simulink model "SubsistemaConRetardo"  (R2024b)
settings: Solver=VariableStepAuto  StartTime=0.0  StopTime=40000  RelTol=1e-3
undefined symbols (not defined in the file): n, p1, p2, p3, Vi
libraries: slpidlib x2, eeAlternativeControllers x1
settings Model: Creator=HP  LastModifiedBy=HP

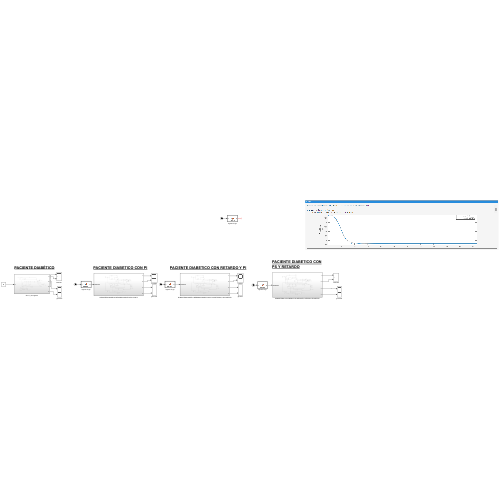
[thumbnail: Simulink's stored preview of the top-level diagram]
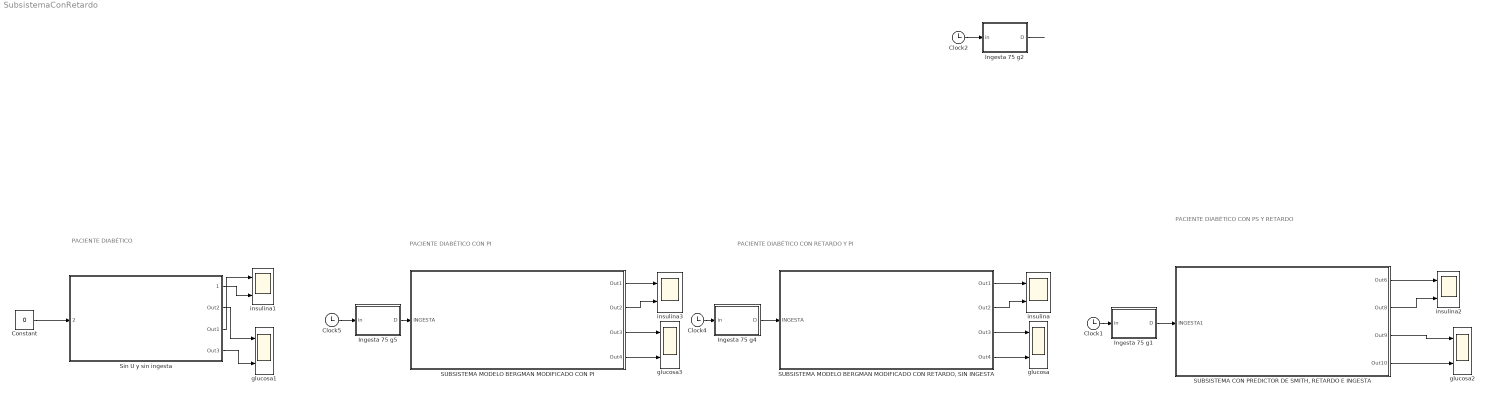
== system SubsistemaConRetardo ==
  note: PACIENTE DIABÉTICO
  note: PACIENTE DIABÉTICO CON RETARDO Y PI
  note: PACIENTE DIABÉTICO CON PI
  note: PACIENTE DIABÉTICO CON PS Y RETARDO
  Clock{1..2,4..5} (4 alike) : Clock
  Constant : Constant  Value=0
  Ingesta 75 g1 : MATLAB Function  TreatAsAtomicUnit=on
  Ingesta 75 g2 : MATLAB Function  TreatAsAtomicUnit=on
  Ingesta 75 g4 : MATLAB Function  TreatAsAtomicUnit=on
  Ingesta 75 g5 : MATLAB Function  TreatAsAtomicUnit=on
  "SUBSISTEMA CON PREDICTOR DE SMITH, RETARDO E INGESTA" : Subsystem
  SUBSISTEMA MODELO BERGMAN MODIFICADO CON PI : Subsystem
  "SUBSISTEMA MODELO BERGMAN MODIFICADO CON RETARDO, SIN INGESTA" : Subsystem
  Sin U y sin ingesta : Subsystem
  glucosa{,1..3} (4 alike) : Scope  NumInputPorts=2
  insulina{,1..3} (4 alike) : Scope  NumInputPorts=2
  wires:
  "SUBSISTEMA MODELO BERGMAN MODIFICADO CON RETARDO, SIN INGESTA"/1(Out1) -> insulina/1
  "SUBSISTEMA MODELO BERGMAN MODIFICADO CON RETARDO, SIN INGESTA"/2(Out2) -> insulina/2
  "SUBSISTEMA MODELO BERGMAN MODIFICADO CON RETARDO, SIN INGESTA"/3(Out3) -> glucosa/1
  "SUBSISTEMA MODELO BERGMAN MODIFICADO CON RETARDO, SIN INGESTA"/4(Out4) -> glucosa/2
  "SUBSISTEMA CON PREDICTOR DE SMITH, RETARDO E INGESTA"/4(Out10) -> glucosa2/2
  "SUBSISTEMA CON PREDICTOR DE SMITH, RETARDO E INGESTA"/2(Out8) -> insulina2/2
  "SUBSISTEMA CON PREDICTOR DE SMITH, RETARDO E INGESTA"/1(Out6) -> insulina2/1
  "SUBSISTEMA CON PREDICTOR DE SMITH, RETARDO E INGESTA"/3(Out9) -> glucosa2/1
  SUBSISTEMA MODELO BERGMAN MODIFICADO CON PI/3(Out3) -> glucosa3/1
  SUBSISTEMA MODELO BERGMAN MODIFICADO CON PI/1(Out1) -> insulina3/1
  SUBSISTEMA MODELO BERGMAN MODIFICADO CON PI/2(Out2) -> insulina3/2
  SUBSISTEMA MODELO BERGMAN MODIFICADO CON PI/4(Out4) -> glucosa3/2
  Sin U y sin ingesta/1(1) -> insulina1/2
  Sin U y sin ingesta/2(Out2) -> glucosa1/1
  Sin U y sin ingesta/3(Out1) -> insulina1/1
  Sin U y sin ingesta/4(Out3) -> glucosa1/2
  Constant/1 -> Sin U y sin ingesta/1(2)
  Ingesta 75 g2/1(D) -> ?
  Clock2/1 -> Ingesta 75 g2/1(in)
  Clock4/1 -> Ingesta 75 g4/1(in)
  Ingesta 75 g4/1(D) -> "SUBSISTEMA MODELO BERGMAN MODIFICADO CON RETARDO, SIN INGESTA"/1(INGESTA)
  Clock5/1 -> Ingesta 75 g5/1(in)
  Ingesta 75 g5/1(D) -> SUBSISTEMA MODELO BERGMAN MODIFICADO CON PI/1(INGESTA)
  Ingesta 75 g1/1(D) -> "SUBSISTEMA CON PREDICTOR DE SMITH, RETARDO E INGESTA"/1(INGESTA1)
  Clock1/1 -> Ingesta 75 g1/1(in)

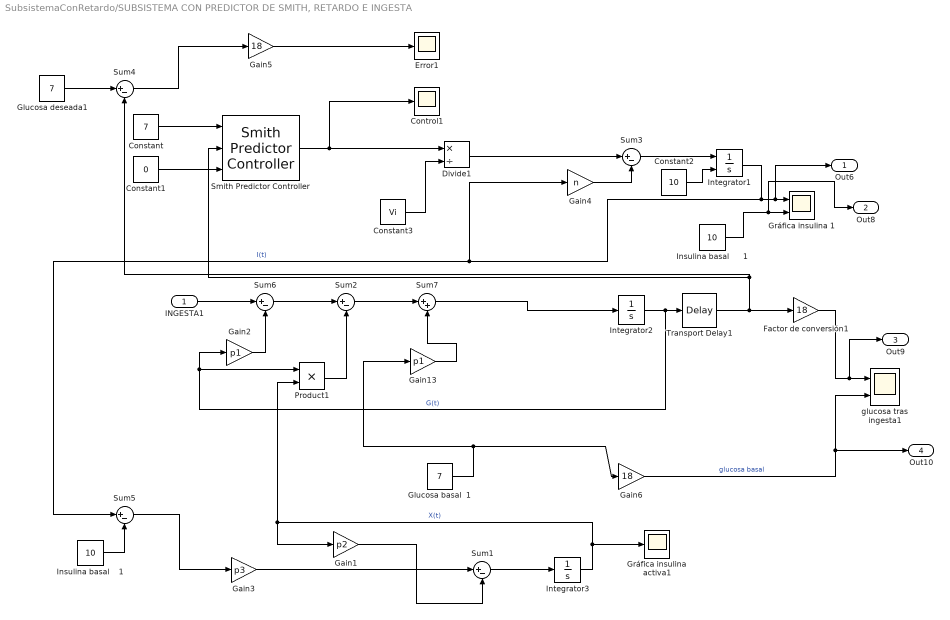
== system SubsistemaConRetardo/SUBSISTEMA CON PREDICTOR DE SMITH, RETARDO E INGESTA ==
  INGESTA1 : Inport
  Constant : Constant  Value=7
  Constant1 : Constant  Value=0
  Constant2 : Constant  Value=10
  Constant3 : Constant  Value=Vi
  Control1 : Scope
  Divide1 : Product  Inputs=*/
  Error1 : Scope
  Factor de conversión1 : Gain  Gain=18
  Gain1 : Gain  Gain=p2
  Gain13 : Gain  Gain=p1
  Gain2 : Gain  Gain=p1
  Gain3 : Gain  Gain=p3
  Gain4 : Gain  Gain=n
  Gain5 : Gain  Gain=18
  Gain6 : Gain  Gain=18
  Glucosa basal  1 : Constant  Value=7
  Glucosa deseada1 : Constant  Value=7
  Gráfica insulina 1 : Scope  NumInputPorts=2
  Gráfica insulina activa1 : Scope
  Insulina basal      1 : Constant  Value=10
  Insulina basal    1 : Constant  Value=10
  Integrator1 : Integrator  InitialConditionSource=external
  Integrator2 : Integrator  InitialCondition=7
  Integrator3 : Integrator
  Product1 : Product
  Smith Predictor Controller : eeAlternativeControllers/Smith Predictor Controller  Kp=-0.3195  Ki=-0.3195/2998.95  x0=0  B=5  A=0  numd=[8.979]  dend=[1, 0.6205, 0.1686]  d=900  Ts=1
  Sum{1..6} (6 alike) : Sum  Inputs=|+-
  Sum7 : Sum  Inputs=|++
  Transport Delay1 : TransportDelay  DelayTime=900  InitialOutput=7
  glucosa tras ingesta1 : Scope  NumInputPorts=2
  Out6 : Outport
  Out8 : Outport  Port=2
  Out9 : Outport  Port=3
  Out10 : Outport  Port=4
  wires:
  Gain13/1 -> Sum7/2
  INGESTA1/1 -> Sum6/1
  Gain2/1 -> Sum6/2
  Sum6/1 -> Sum2/1
  Insulina basal      1/1 -> Out8/1, Gráfica insulina 1/2
  Gain4/1 -> Sum3/2
  Integrator1/1 -> Out6/1, Gráfica insulina 1/1, Sum5/1, Gain4/1  "I(t)"
  Gain5/1 -> Error1/1
  Factor de conversión1/1 -> Out9/1, glucosa tras ingesta1/1
  Sum7/1 -> Integrator2/1
  Sum5/1 -> Gain3/1
  Sum3/1 -> Integrator1/1
  Sum4/1 -> Gain5/1
  Product1/1 -> Sum2/2
  Constant3/1 -> Divide1/2
  Integrator3/1 -> Product1/2, Gain1/1, Gráfica insulina activa1/1  "X(t)"
  Gain6/1 -> Out10/1, glucosa tras ingesta1/2  "glucosa basal"
  Glucosa deseada1/1 -> Sum4/1
  Integrator2/1 -> Gain2/1, Product1/1, Transport Delay1/1  "G(t)"
  Glucosa basal  1/1 -> Gain13/1, Gain6/1
  Divide1/1 -> Sum3/1
  Constant2/1 -> Integrator1/2
  Sum2/1 -> Sum7/1
  Smith Predictor Controller/1 -> Control1/1, Divide1/1
  Gain1/1 -> Sum1/2
  Constant1/1 -> Smith Predictor Controller/3
  Insulina basal    1/1 -> Sum5/2
  Gain3/1 -> Sum1/1
  Constant/1 -> Smith Predictor Controller/1
  Sum1/1 -> Integrator3/1
  Transport Delay1/1 -> Smith Predictor Controller/2, Sum4/2, Factor de conversión1/1

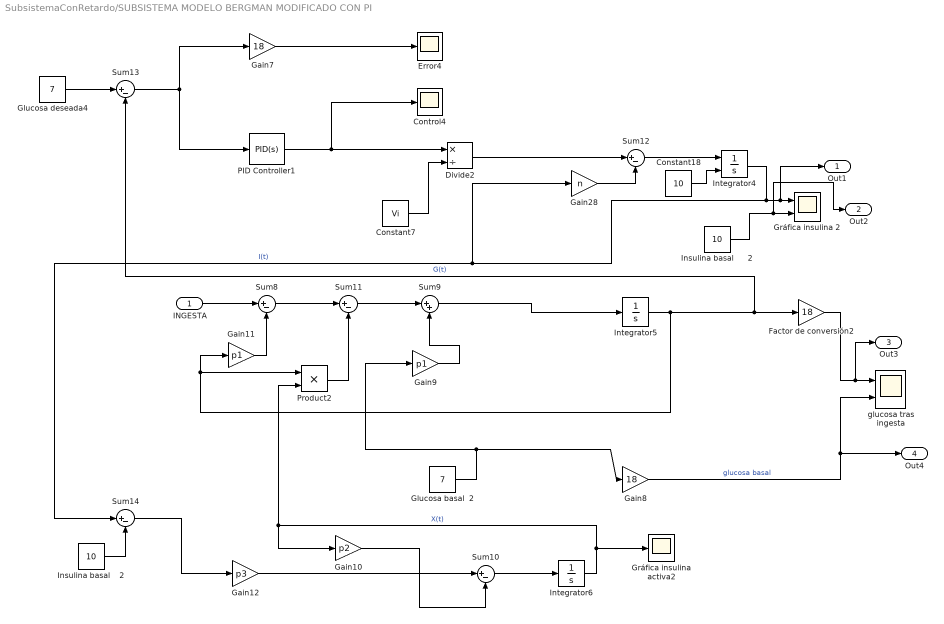
== system SubsistemaConRetardo/SUBSISTEMA MODELO BERGMAN MODIFICADO CON PI ==
  INGESTA : Inport
  Constant18 : Constant  Value=10
  Constant7 : Constant  Value=Vi
  Control4 : Scope
  Divide2 : Product  Inputs=*/
  Error4 : Scope
  Factor de conversión2 : Gain  Gain=18
  Gain10 : Gain  Gain=p2
  Gain11 : Gain  Gain=p1
  Gain12 : Gain  Gain=p3
  Gain28 : Gain  Gain=n
  Gain7 : Gain  Gain=18
  Gain8 : Gain  Gain=18
  Gain9 : Gain  Gain=p1
  Glucosa basal  2 : Constant  Value=7
  Glucosa deseada4 : Constant  Value=7
  Gráfica insulina 2 : Scope  NumInputPorts=2
  Gráfica insulina activa2 : Scope
  Insulina basal      2 : Constant  Value=10
  Insulina basal    2 : Constant  Value=10
  Integrator4 : Integrator  InitialConditionSource=external
  Integrator5 : Integrator  InitialCondition=7
  Integrator6 : Integrator
  PID Controller1 : slpidlib/PID Controller  Controller=PID  Form=Parallel  TimeDomain=Continuous-time  UseExternalTs=off  SampleTime=-1  IntegratorMethod=Forward Euler  FilterMethod=Forward Euler  ControllerParametersSource=internal  P=-0.3195  I=-0.3195/2998.95  UseKiTs=off  D=0  UseExternalDerivativeSource=off  N=10  UseFilter=on  TunerSelectOption=Transfer Function Based (PID Tuner App)  InitialConditionSource=internal  InitialConditionForIntegrator=0  InitialConditionForFilter=0  DifferentiatorICPrevScaledInput=0  ExternalReset=none  TrackingMode=off  Kt=1  LimitOutput=off  SatLimitsSource=internal  UpperSaturationLimit=inf  LowerSaturationLimit=-inf  LinearizeAsGain=on  AntiWindupMode=none  Kb=1  LimitIntegrator=off  UpperIntegratorSaturationLimit=inf  LowerIntegratorSaturationLimit=-inf  POutMin=[]  POutMax=[]  IOutMin=[]  IOutMax=[]  DOutMin=[]  DOutMax=[]  NOutMin=[]  NOutMax=[]  SumOutMin=[]  SumOutMax=[]  SaturationOutMin=[]  SaturationOutMax=[]  PParamMin=[]  PParamMax=[]  IParamMin=[]  IParamMax=[]  DParamMin=[]  DParamMax=[]  NParamMin=[]  NParamMax=[]  KbParamMin=[]  KbParamMax=[]  KtParamMin=[]  KtParamMax=[]  KbOutMin=[]  KbOutMax=[]  KtOutMin=[]  KtOutMax=[]  IntegratorOutMin=[]  IntegratorOutMax=[]  FilterOutMin=[]  FilterOutMax=[]  SumI1OutMin=[]  SumI1OutMax=[]  SumI2OutMin=[]  SumI2OutMax=[]  SumI3OutMin=[]  SumI3OutMax=[]  SumI4OutMin=[]  SumI4OutMax=[]  SumDOutMin=[]  SumDOutMax=[]  DifferentiatorOutMin=[]  DifferentiatorOutMax=[]  FilterDiffOutCoefMin=[]  FilterDiffOutCoefMax=[]  ReciprocalOutMin=[]  ReciprocalOutMax=[]  SumDenOutMin=[]  SumDenOutMax=[]  SumNumOutMin=[]  SumNumOutMax=[]  DivideOutMin=[]  DivideOutMax=[]  UdiffTsProdOutMin=[]  UdiffTsProdOutMax=[]  NTsProdOutMin=[]  NTsProdOutMax=[]  UintegralTsProdOutMin=[]  UintegralTsProdOutMax=[]  UngainTsProdOutMin=[]  UngainTsProdOutMax=[]  ClampingZeroOutDataTypeStr=Inherit: Inherit via back propagation  ClampingZeroOutMin=[]  ClampingZeroOutMax=[]  FilterDenConstantOutDataTypeStr=Inherit: Inherit via back propagation  FilterDenConstantOutMin=[]  FilterDenConstantOutMax=[]  PCopyOutDataTypeStr=Inherit: Inherit via back propagation  PCopyOutMin=[]  PCopyOutMax=[]  NCopyOutDataTypeStr=Inherit: Inherit via back propagation  NCopyOutMin=[]  NCopyOutMax=[]  IntegratorContinuousStateAttributes=''  IntegratorStateMustResolveToSignalObject=off  IntegratorRTWStateStorageClass=Auto  FilterContinuousStateAttributes=''  FilterStateMustResolveToSignalObject=off  FilterRTWStateStorageClass=Auto  ParallelPVariant=InternalParameters  IdealPVariant=Disabled  IVariant=InternalParameters  DVariant=InternalParameters  IntegratorVariant=Continuous  SatVariant=Disabled  AWVariant=Passthrough  PCopyVariant=Disabled  TRVariant=Disabled  FdbkBlocksVariant=Forward  IdealPFdbkVariant=Disabled  SatFdbkVariant=Disabled  DerivativeFilterVariant=ContFilter  NVariant=InternalParameters  NCopyVariant=Disabled  FilterICVariant=InternalICsFilter  IntegratorICVariant=InternalICs  ExternalResetVariant=Disabled  TRSumVariant=Passthrough  SumFdbkVariant=Disabled  SumVariant=Sum_PID  TsampFilterVariant=InternalTs  TsampNgainVariant=Passthrough  TsampIntegralVariant=Disabled_SignalSpec  ExternalSaturationOutDataTypeStr=Inherit: Same as second input  DerivativeSourceVariant=ErrorSignal  PreIntVariant=InternalPreInt
  Product2 : Product
  Sum{8,10..14} (6 alike) : Sum  Inputs=|+-
  Sum9 : Sum  Inputs=|++
  glucosa tras ingesta : Scope  NumInputPorts=2
  Out1 : Outport
  Out2 : Outport  Port=2
  Out3 : Outport  Port=3
  Out4 : Outport  Port=4
  wires:
  Integrator6/1 -> Product2/2, Gain10/1, Gráfica insulina activa2/1  "X(t)"
  Factor de conversión2/1 -> Out3/1, glucosa tras ingesta/1
  Sum11/1 -> Sum9/1
  Sum12/1 -> Integrator4/1
  Integrator5/1 -> Sum13/2, Factor de conversión2/1, Gain11/1, Product2/1  "G(t)"
  Gain8/1 -> glucosa tras ingesta/2, Out4/1  "glucosa basal"
  Sum14/1 -> Gain12/1
  Insulina basal      2/1 -> Out2/1, Gráfica insulina 2/2
  Integrator4/1 -> Out1/1, Gráfica insulina 2/1, Sum14/1, Gain28/1  "I(t)"
  Gain9/1 -> Sum9/2
  Glucosa basal  2/1 -> Gain9/1, Gain8/1
  Gain12/1 -> Sum10/1
  Glucosa deseada4/1 -> Sum13/1
  Constant7/1 -> Divide2/2
  Sum9/1 -> Integrator5/1
  Gain10/1 -> Sum10/2
  Product2/1 -> Sum11/2
  Gain28/1 -> Sum12/2
  Sum10/1 -> Integrator6/1
  Sum8/1 -> Sum11/1
  Sum13/1 -> PID Controller1/1, Gain7/1
  Insulina basal    2/1 -> Sum14/2
  Gain11/1 -> Sum8/2
  Gain7/1 -> Error4/1
  Divide2/1 -> Sum12/1
  PID Controller1/1 -> Control4/1, Divide2/1
  Constant18/1 -> Integrator4/2
  INGESTA/1 -> Sum8/1

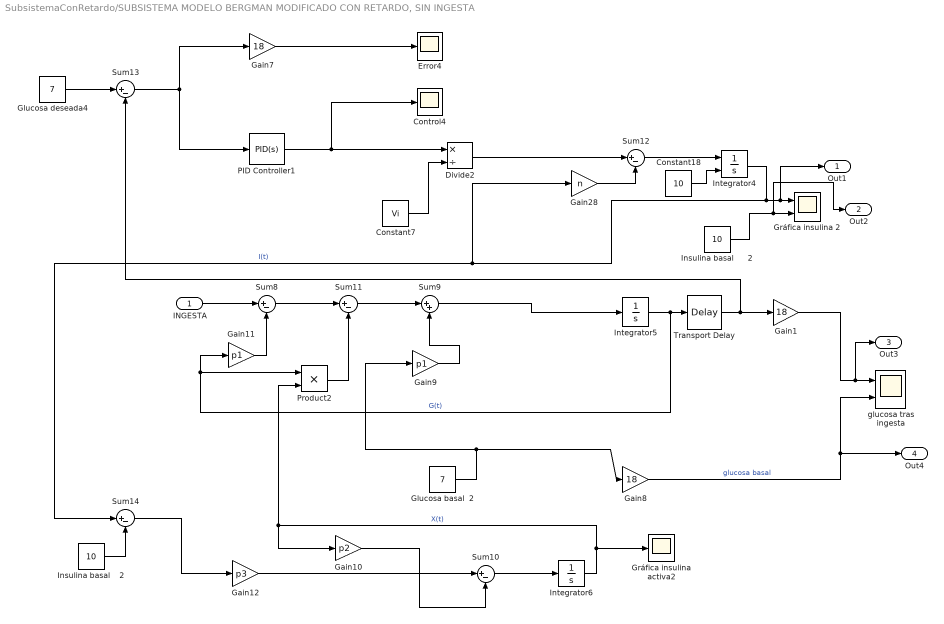
== system SubsistemaConRetardo/SUBSISTEMA MODELO BERGMAN MODIFICADO CON RETARDO, SIN INGESTA ==
  INGESTA : Inport
  Constant18 : Constant  Value=10
  Constant7 : Constant  Value=Vi
  Control4 : Scope
  Divide2 : Product  Inputs=*/
  Error4 : Scope
  Gain1 : Gain  Gain=18
  Gain10 : Gain  Gain=p2
  Gain11 : Gain  Gain=p1
  Gain12 : Gain  Gain=p3
  Gain28 : Gain  Gain=n
  Gain7 : Gain  Gain=18
  Gain8 : Gain  Gain=18
  Gain9 : Gain  Gain=p1
  Glucosa basal  2 : Constant  Value=7
  Glucosa deseada4 : Constant  Value=7
  Gráfica insulina 2 : Scope  NumInputPorts=2
  Gráfica insulina activa2 : Scope
  Insulina basal      2 : Constant  Value=10
  Insulina basal    2 : Constant  Value=10
  Integrator4 : Integrator  InitialConditionSource=external
  Integrator5 : Integrator  InitialCondition=7
  Integrator6 : Integrator
  PID Controller1 : slpidlib/PID Controller  Controller=PID  Form=Parallel  TimeDomain=Continuous-time  UseExternalTs=off  SampleTime=-1  IntegratorMethod=Forward Euler  FilterMethod=Forward Euler  ControllerParametersSource=internal  P=-0.3195  I=-0.3195/2998.95  UseKiTs=off  D=0  UseExternalDerivativeSource=off  N=10  UseFilter=on  TunerSelectOption=Transfer Function Based (PID Tuner App)  InitialConditionSource=internal  InitialConditionForIntegrator=0  InitialConditionForFilter=0  DifferentiatorICPrevScaledInput=0  ExternalReset=none  TrackingMode=off  Kt=1  LimitOutput=off  SatLimitsSource=internal  UpperSaturationLimit=inf  LowerSaturationLimit=-inf  LinearizeAsGain=on  AntiWindupMode=none  Kb=1  LimitIntegrator=off  UpperIntegratorSaturationLimit=inf  LowerIntegratorSaturationLimit=-inf  POutMin=[]  POutMax=[]  IOutMin=[]  IOutMax=[]  DOutMin=[]  DOutMax=[]  NOutMin=[]  NOutMax=[]  SumOutMin=[]  SumOutMax=[]  SaturationOutMin=[]  SaturationOutMax=[]  PParamMin=[]  PParamMax=[]  IParamMin=[]  IParamMax=[]  DParamMin=[]  DParamMax=[]  NParamMin=[]  NParamMax=[]  KbParamMin=[]  KbParamMax=[]  KtParamMin=[]  KtParamMax=[]  KbOutMin=[]  KbOutMax=[]  KtOutMin=[]  KtOutMax=[]  IntegratorOutMin=[]  IntegratorOutMax=[]  FilterOutMin=[]  FilterOutMax=[]  SumI1OutMin=[]  SumI1OutMax=[]  SumI2OutMin=[]  SumI2OutMax=[]  SumI3OutMin=[]  SumI3OutMax=[]  SumI4OutMin=[]  SumI4OutMax=[]  SumDOutMin=[]  SumDOutMax=[]  DifferentiatorOutMin=[]  DifferentiatorOutMax=[]  FilterDiffOutCoefMin=[]  FilterDiffOutCoefMax=[]  ReciprocalOutMin=[]  ReciprocalOutMax=[]  SumDenOutMin=[]  SumDenOutMax=[]  SumNumOutMin=[]  SumNumOutMax=[]  DivideOutMin=[]  DivideOutMax=[]  UdiffTsProdOutMin=[]  UdiffTsProdOutMax=[]  NTsProdOutMin=[]  NTsProdOutMax=[]  UintegralTsProdOutMin=[]  UintegralTsProdOutMax=[]  UngainTsProdOutMin=[]  UngainTsProdOutMax=[]  ClampingZeroOutDataTypeStr=Inherit: Inherit via back propagation  ClampingZeroOutMin=[]  ClampingZeroOutMax=[]  FilterDenConstantOutDataTypeStr=Inherit: Inherit via back propagation  FilterDenConstantOutMin=[]  FilterDenConstantOutMax=[]  PCopyOutDataTypeStr=Inherit: Inherit via back propagation  PCopyOutMin=[]  PCopyOutMax=[]  NCopyOutDataTypeStr=Inherit: Inherit via back propagation  NCopyOutMin=[]  NCopyOutMax=[]  IntegratorContinuousStateAttributes=''  IntegratorStateMustResolveToSignalObject=off  IntegratorRTWStateStorageClass=Auto  FilterContinuousStateAttributes=''  FilterStateMustResolveToSignalObject=off  FilterRTWStateStorageClass=Auto  ParallelPVariant=InternalParameters  IdealPVariant=Disabled  IVariant=InternalParameters  DVariant=InternalParameters  IntegratorVariant=Continuous  SatVariant=Disabled  AWVariant=Passthrough  PCopyVariant=Disabled  TRVariant=Disabled  FdbkBlocksVariant=Forward  IdealPFdbkVariant=Disabled  SatFdbkVariant=Disabled  DerivativeFilterVariant=ContFilter  NVariant=InternalParameters  NCopyVariant=Disabled  FilterICVariant=InternalICsFilter  IntegratorICVariant=InternalICs  ExternalResetVariant=Disabled  TRSumVariant=Passthrough  SumFdbkVariant=Disabled  SumVariant=Sum_PID  TsampFilterVariant=InternalTs  TsampNgainVariant=Passthrough  TsampIntegralVariant=Disabled_SignalSpec  ExternalSaturationOutDataTypeStr=Inherit: Same as second input  DerivativeSourceVariant=ErrorSignal  PreIntVariant=InternalPreInt
  Product2 : Product
  Sum{8,10..14} (6 alike) : Sum  Inputs=|+-
  Sum9 : Sum  Inputs=|++
  Transport Delay : TransportDelay  DelayTime=900  InitialOutput=7
  glucosa tras ingesta : Scope  NumInputPorts=2
  Out1 : Outport
  Out2 : Outport  Port=2
  Out3 : Outport  Port=3
  Out4 : Outport  Port=4
  wires:
  Integrator6/1 -> Product2/2, Gain10/1, Gráfica insulina activa2/1  "X(t)"
  Transport Delay/1 -> Sum13/2, Gain1/1
  Sum11/1 -> Sum9/1
  Sum12/1 -> Integrator4/1
  Integrator5/1 -> Gain11/1, Product2/1, Transport Delay/1  "G(t)"
  Gain8/1 -> glucosa tras ingesta/2, Out4/1  "glucosa basal"
  Sum14/1 -> Gain12/1
  Insulina basal      2/1 -> Out2/1, Gráfica insulina 2/2
  Integrator4/1 -> Out1/1, Gráfica insulina 2/1, Sum14/1, Gain28/1  "I(t)"
  Gain9/1 -> Sum9/2
  Glucosa basal  2/1 -> Gain9/1, Gain8/1
  Gain12/1 -> Sum10/1
  Glucosa deseada4/1 -> Sum13/1
  Constant7/1 -> Divide2/2
  Sum9/1 -> Integrator5/1
  Gain10/1 -> Sum10/2
  Product2/1 -> Sum11/2
  Gain28/1 -> Sum12/2
  Sum10/1 -> Integrator6/1
  Sum8/1 -> Sum11/1
  Sum13/1 -> PID Controller1/1, Gain7/1
  Insulina basal    2/1 -> Sum14/2
  Gain11/1 -> Sum8/2
  Gain7/1 -> Error4/1
  Divide2/1 -> Sum12/1
  PID Controller1/1 -> Control4/1, Divide2/1
  Constant18/1 -> Integrator4/2
  INGESTA/1 -> Sum8/1
  Gain1/1 -> Out3/1, glucosa tras ingesta/1

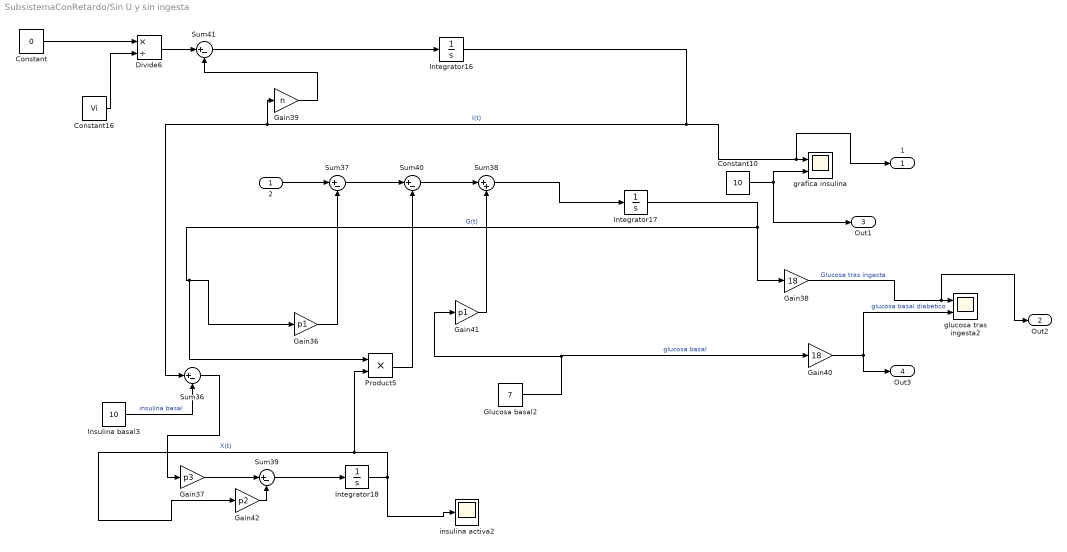
== system SubsistemaConRetardo/Sin U y sin ingesta ==
  2 : Inport
  Constant : Constant  Value=0
  Constant10 : Constant  Value=10
  Constant16 : Constant  Value=Vi
  Divide6 : Product  Inputs=*/
  Gain36 : Gain  Gain=p1
  Gain37 : Gain  Gain=p3
  Gain38 : Gain  Gain=18
  Gain39 : Gain  Gain=n
  Gain40 : Gain  Gain=18
  Gain41 : Gain  Gain=p1
  Gain42 : Gain  Gain=p2
  Glucosa basal2 : Constant  Value=7
  Insulina basal3 : Constant  Value=10
  Integrator16 : Integrator  InitialCondition=10
  Integrator17 : Integrator  InitialCondition=7
  Integrator18 : Integrator
  Product5 : Product
  Sum{36..37,39..41} (5 alike) : Sum  Inputs=|+-
  Sum38 : Sum  Inputs=|++
  glucosa tras ingesta2 : Scope  NumInputPorts=2
  grafica insulina : Scope  NumInputPorts=2
  insulina activa2 : Scope
  1 : Outport
  Out2 : Outport  Port=2
  Out1 : Outport  Port=3
  Out3 : Outport  Port=4
  wires:
  Integrator18/1 -> insulina activa2/1, Product5/2, Gain42/1  "X(t)"
  Integrator17/1 -> Gain38/1, Product5/1, Gain36/1  "G(t)"
  Gain39/1 -> Sum41/2
  Glucosa basal2/1 -> Gain41/1, Gain40/1  "glucosa basal"
  Integrator16/1 -> Sum36/1, Gain39/1, 1/1, grafica insulina/1  "I(t)"
  Constant10/1 -> Out1/1, grafica insulina/2
  Gain42/1 -> Sum39/2
  2/1 -> Sum37/1
  Sum37/1 -> Sum40/1
  Sum39/1 -> Integrator18/1
  Gain40/1 -> glucosa tras ingesta2/2, Out3/1  "glucosa basal diabetico"
  Sum40/1 -> Sum38/1
  Constant/1 -> Divide6/1
  Gain36/1 -> Sum37/2
  Gain38/1 -> Out2/1, glucosa tras ingesta2/1  "Glucosa tras ingesta"
  Sum36/1 -> Gain37/1
  Gain41/1 -> Sum38/2
  Gain37/1 -> Sum39/1
  Sum41/1 -> Integrator16/1
  Sum38/1 -> Integrator17/1
  Insulina basal3/1 -> Sum36/2  "insulina basal"
  Divide6/1 -> Sum41/1
  Constant16/1 -> Divide6/2
  Product5/1 -> Sum40/2

== matlab function SubsistemaConRetardo/Ingesta 75 g2 ==
  data: in input; D output
function D = comida(in)
% Variables de entrada en la funcion
t = in(1) %- 8*60*60; % Ajuste para iniciar a las 8 de la mañana
 
% Parámetros del modelo
Ag = 0.8; % adimensional
Tmaxi = 55*60; % s
Vg = 13.79; % L
Tmaxg = 40*60; % s
t1 = 0;
Dg = 0;
f = 1000/180; % factor de conversión de g a mmol
 
% Comidas (perturbaciones) a lo largo de un día
Dg = 50*f;
% Ecuación
D = (Dg*Ag*(t-t1)*exp(-(t-t1)/Tmaxi))/(Vg*Tmaxg^2);

== matlab function SubsistemaConRetardo/Ingesta 75 g4 ==
  data: in input; D output
function D = comida(in)
% Variables de entrada en la funcion
t = in(1) %- 8*60*60; % Ajuste para iniciar a las 8 de la mañana
 
% Parámetros del modelo
Ag = 0.8; % adimensional
Tmaxi = 55*60; % s
Vg = 13.79; % L
Tmaxg = 40*60; % s
t1 = 0;
Dg = 0;
f = 1000/180; % factor de conversión de g a mmol
 
% Comidas (perturbaciones) a lo largo de un día
Dg = 50*f;
% Ecuación
D = (Dg*Ag*(t-t1)*exp(-(t-t1)/Tmaxi))/(Vg*Tmaxg^2);

== matlab function SubsistemaConRetardo/Ingesta 75 g5 ==
  data: in input; D output
function D = comida(in)
% Variables de entrada en la funcion
t = in(1) %- 8*60*60; % Ajuste para iniciar a las 8 de la mañana
 
% Parámetros del modelo
Ag = 0.8; % adimensional
Tmaxi = 55*60; % s
Vg = 13.79; % L
Tmaxg = 40*60; % s
t1 = 0;
Dg = 0;
f = 1000/180; % factor de conversión de g a mmol
 
% Comidas (perturbaciones) a lo largo de un día
Dg = 50*f;
% Ecuación
D = (Dg*Ag*(t-t1)*exp(-(t-t1)/Tmaxi))/(Vg*Tmaxg^2);

== matlab function SubsistemaConRetardo/Ingesta 75 g1 ==
  data: in input; D output
function D = comida(in)
% Variables de entrada en la funcion
t = in(1) %- 8*60*60; % Ajuste para iniciar a las 8 de la mañana
 
% Parámetros del modelo
Ag = 0.8; % adimensional
Tmaxi = 55*60; % s
Vg = 13.79; % L
Tmaxg = 40*60; % s
t1 = 0;
Dg = 0;
f = 1000/180; % factor de conversión de g a mmol
 
% Comidas (perturbaciones) a lo largo de un día
Dg = 50*f;
% Ecuación
D = (Dg*Ag*(t-t1)*exp(-(t-t1)/Tmaxi))/(Vg*Tmaxg^2);
